simulink model "newPID"  (R2023b)
settings: Solver=VariableStepAuto  StartTime=0.0  StopTime=10.0  RelTol=1e-3
libraries: simulink x3, slpidlib x2
settings Model: Creator=Penis  LastModifiedBy=Alex
settings RTWCC: GPUComputeCapability=5.0

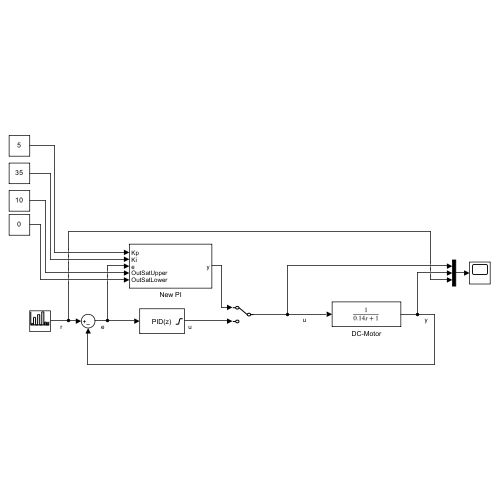
[thumbnail: Simulink's stored preview of the top-level diagram]
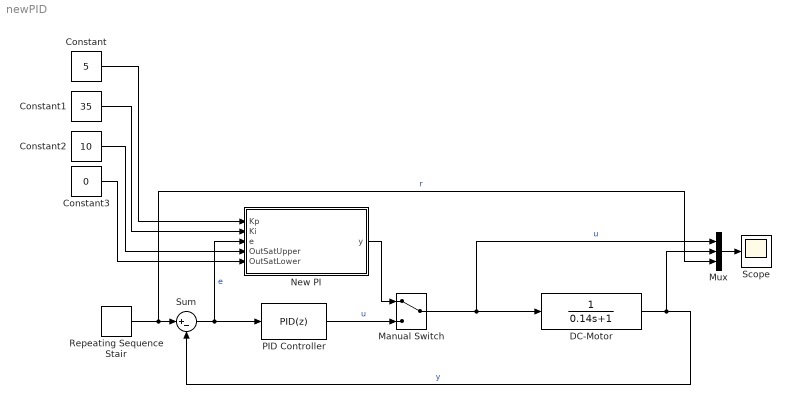
== system newPID ==
  Constant : Constant  Value=5
  Constant1 : Constant  Value=35
  Constant2 : Constant  Value=10
  Constant3 : Constant  Value=0
  DC-Motor : TransferFcn  Denominator=[0.14 1]
  Manual Switch : ManualSwitch
  Mux : Mux  Inputs=3
  New PI : Subsystem
  PID Controller : slpidlib/PID Controller  Controller=PID  Form=Parallel  TimeDomain=Discrete-time  UseExternalTs=off  SampleTime=0.01  IntegratorMethod=Forward Euler  FilterMethod=Forward Euler  ControllerParametersSource=internal  P=5  I=35  UseKiTs=off  D=0  N=0  UseFilter=on  TunerSelectOption=Transfer Function Based (PID Tuner App)  InitialConditionSource=internal  InitialConditionForIntegrator=0  InitialConditionForFilter=0  DifferentiatorICPrevScaledInput=0  ExternalReset=none  TrackingMode=off  Kt=1  LimitOutput=on  SatLimitsSource=internal  UpperSaturationLimit=10  LowerSaturationLimit=0  LinearizeAsGain=on  AntiWindupMode=clamping  Kb=1  LimitIntegrator=on  UpperIntegratorSaturationLimit=10  LowerIntegratorSaturationLimit=-10  POutMin=[]  POutMax=[]  IOutMin=[]  IOutMax=[]  DOutMin=[]  DOutMax=[]  NOutMin=[]  NOutMax=[]  SumOutMin=[]  SumOutMax=[]  SaturationOutMin=[]  SaturationOutMax=[]  PParamMin=[]  PParamMax=[]  IParamMin=[]  IParamMax=[]  DParamMin=[]  DParamMax=[]  NParamMin=[]  NParamMax=[]  KbParamMin=[]  KbParamMax=[]  KtParamMin=[]  KtParamMax=[]  KbOutMin=[]  KbOutMax=[]  KtOutMin=[]  KtOutMax=[]  IntegratorOutMin=[]  IntegratorOutMax=[]  FilterOutMin=[]  FilterOutMax=[]  SumI1OutMin=[]  SumI1OutMax=[]  SumI2OutMin=[]  SumI2OutMax=[]  SumI3OutMin=[]  SumI3OutMax=[]  SumI4OutMin=[]  SumI4OutMax=[]  SumDOutMin=[]  SumDOutMax=[]  DifferentiatorOutMin=[]  DifferentiatorOutMax=[]  FilterDiffOutCoefMin=[]  FilterDiffOutCoefMax=[]  ReciprocalOutMin=[]  ReciprocalOutMax=[]  SumDenOutMin=[]  SumDenOutMax=[]  SumNumOutMin=[]  SumNumOutMax=[]  DivideOutMin=[]  DivideOutMax=[]  UdiffTsProdOutMin=[]  UdiffTsProdOutMax=[]  NTsProdOutMin=[]  NTsProdOutMax=[]  UintegralTsProdOutMin=[]  UintegralTsProdOutMax=[]  UngainTsProdOutMin=[]  UngainTsProdOutMax=[]  ClampingZeroOutDataTypeStr=Inherit: Inherit via back propagation  ClampingZeroOutMin=[]  ClampingZeroOutMax=[]  FilterDenConstantOutDataTypeStr=Inherit: Inherit via back propagation  FilterDenConstantOutMin=[]  FilterDenConstantOutMax=[]  PCopyOutDataTypeStr=Inherit: Inherit via back propagation  PCopyOutMin=[]  PCopyOutMax=[]  NCopyOutDataTypeStr=Inherit: Inherit via back propagation  NCopyOutMin=[]  NCopyOutMax=[]  IntegratorContinuousStateAttributes=''  IntegratorStateMustResolveToSignalObject=off  IntegratorRTWStateStorageClass=Auto  FilterContinuousStateAttributes=''  FilterStateMustResolveToSignalObject=off  FilterRTWStateStorageClass=Auto  ParallelPVariant=InternalParameters  IdealPVariant=Disabled  IVariant=InternalParameters  DVariant=InternalParameters  IntegratorVariant=Discrete  SatVariant=Enabled  AWVariant=DiscClampingParallel  PCopyVariant=Disabled  TRVariant=Disabled  FdbkBlocksVariant=Forward  IdealPFdbkVariant=Disabled  SatFdbkVariant=Disabled  DerivativeFilterVariant=ForwardEulerFilter  NVariant=InternalParameters  NCopyVariant=Disabled  FilterICVariant=InternalICsFilter  IntegratorICVariant=InternalICs  ExternalResetVariant=Disabled  TRSumVariant=Passthrough  SumFdbkVariant=Disabled  SumVariant=Sum_PID  TsampFilterVariant=InternalTs  TsampNgainVariant=Passthrough  TsampIntegralVariant=Disabled_SignalSpec  ExternalSaturationOutDataTypeStr=Inherit: Same as second input
  Repeating Sequence Stair : simulink/Sources/Repeating Sequence Stair  OutValues=[0 1 0 5 5 0 0 7 7 0 0 9 9 0 2 0 2 0 2].'  tsamp=0.5  OutMin=[]  OutMax=[]  OutDataTypeStr=double  OutputDataTypeScalingMode=double  OutDataType=fixdt(0,8)  ConRadixGroup=Best Precision: Vector-wise  OutScaling=2^-12
  Scope : Scope
  Sum : Sum  Inputs=|+-
  wires:
  Manual Switch/1 -> DC-Motor/1, Mux/1  "u"
  Mux/1 -> Scope/1
  DC-Motor/1 -> Sum/2, Mux/2  "y"
  Sum/1 -> New PI/3(e), PID Controller/1  "e"
  Repeating Sequence Stair/1 -> Mux/3, Sum/1  "r"
  PID Controller/1 -> Manual Switch/2  "u"
  New PI/1(y) -> Manual Switch/1
  Constant/1 -> New PI/1(Kp)
  Constant1/1 -> New PI/2(Ki)
  Constant2/1 -> New PI/4(OutSatUpper)
  Constant3/1 -> New PI/5(OutSatLower)

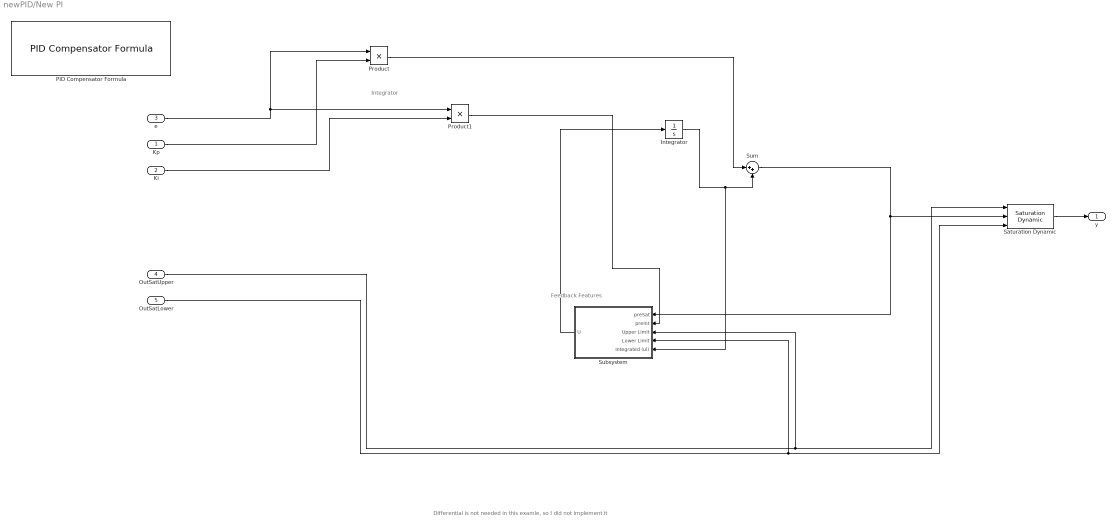
== system newPID/New PI ==
  note: Differential is not needed in this examle, so I did not implement it
  note: Integrator
  note: Feedback Features
  Kp : Inport
  Ki : Inport  Port=2
  e : Inport  Port=3
  OutSatUpper : Inport  Port=4
  OutSatLower : Inport  Port=5
  Integrator : Integrator  LimitOutput=on  UpperSaturationLimit=10  LowerSaturationLimit=-10
  PID Compensator Formula : slpidlib/PID Controller/PID Compensator Formula  SystemSampleTime=-1  VariantActivationTime=update diagram  AllowFlexibleInterface=on  Latency=0  AutoFrameSizeCalculation=off
  Product : Product
  Product1 : Product
  Saturation Dynamic : simulink/Discontinuities/Saturation Dynamic  OutMin=[]  OutMax=[]  OutDataTypeStr=Inherit: Same as second input  OutDataType=fixdt(1, 16)  OutScaling=2^-10  DoSatur=off
  Subsystem : Subsystem
  Sum : Sum  Inputs=|++
  y : Outport  SampleTime=0.01
  wires:
  Integrator/1 -> Sum/2, Subsystem/5(Integrated (ui))
  Subsystem/1(U) -> Integrator/1
  Saturation Dynamic/1 -> y/1
  Sum/1 -> Saturation Dynamic/2, Subsystem/1(preSat)
  e/1 -> Product/1, Product1/1
  Kp/1 -> Product/2
  Product/1 -> Sum/1
  Ki/1 -> Product1/2
  Product1/1 -> Subsystem/2(preInt)
  OutSatUpper/1 -> Subsystem/3(Upper Limit), Saturation Dynamic/1
  OutSatLower/1 -> Subsystem/4(Lower Limit), Saturation Dynamic/3

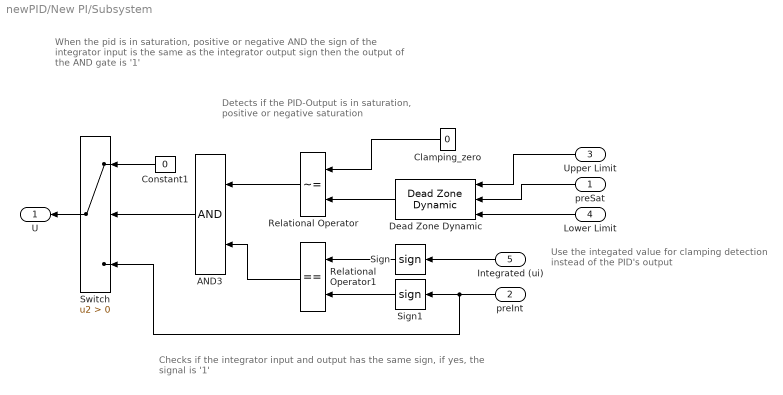
== system newPID/New PI/Subsystem ==
  note: Use the integated value for
      | clamping detection instead of the PID's output
  note: When the pid is in saturation, positive or negative AND
      | the sign of the integrator input is the same as the integrator output sign
      | then the output of the AND gate is '1'
  note: Detects if the PID-Output is in saturation,
      | positive or negative saturation
  note: Checks if the integrator input and output has the same sign,
      | if yes, the signal is '1'
  preSat : Inport
  preInt : Inport  Port=2
  Upper Limit : Inport  Port=3
  Lower Limit : Inport  Port=4
  Integrated (ui) : Inport  Port=5
  AND3 : Logic  DisableCoverage=on  OutDataTypeStr=boolean
  Clamping_zero : Constant  DisableCoverage=on  Value=0  OutMin=0  OutMax=0  OutDataTypeStr=Inherit: Inherit via back propagation
  Constant1 : Constant  DisableCoverage=on  Value=0  OutDataTypeStr=Inherit: Inherit via back propagation  PreserveConstantTs=on
  Dead Zone Dynamic : simulink/Discontinuities/Dead Zone Dynamic
  Relational Operator : RelationalOperator  DisableCoverage=on  Operator=~=  OutDataTypeStr=boolean  RndMeth=Simplest  InputSameDT=off
  Relational Operator1 : RelationalOperator  DisableCoverage=on  Operator===  OutDataTypeStr=boolean  RndMeth=Simplest  InputSameDT=off
  Sign : Signum
  Sign1 : Signum
  Switch : Switch  Criteria=u2 > Threshold  SaturateOnIntegerOverflow=off
  U : Outport
  wires:
  Clamping_zero/1 -> Relational Operator/1
  Upper Limit/1 -> Dead Zone Dynamic/1
  Relational Operator/1 -> AND3/1
  AND3/1 -> Switch/2
  preInt/1 -> Switch/3, Sign1/1
  preSat/1 -> Dead Zone Dynamic/2
  Dead Zone Dynamic/1 -> Relational Operator/2
  Switch/1 -> U/1
  Lower Limit/1 -> Dead Zone Dynamic/3
  Constant1/1 -> Switch/1
  Integrated (ui)/1 -> Sign/1
  Sign/1 -> Relational Operator1/1
  Sign1/1 -> Relational Operator1/2
  Relational Operator1/1 -> AND3/2
